simulink model "HybridControllerD2D2"  (R2017b)
settings: Solver=FixedStepDiscrete  StartTime=0.0  StopTime=inf  FixedStep=controlPeriod  RelTol=1e-3
PreLoadFcn:
  | initializeSimulation
  | initializeSCRAMNet
  | ATS_setup
values from neighbouring files (symbols this model uses):
  controlPeriod = 1/2048    (= 0.00048828125)    [initializeSCRAMNet.m]
  dofID = [1]    [initializeSimulation.m]
  lhpNode = node    [initializeSCRAMNet.m]
  MRC = [2 0.05 0.001]./10    [ATS_setup.m]
  Nl = floor(tl*sample_rate)    [ATS_setup.m]
  nTbl = 1    [initializeSCRAMNet.m]
  opfNode = node    [initializeSCRAMNet.m]
  P_range = [0.9 1.1 ... (first row only)    [ATS_setup.m]
  sample = 1/2048    (= 0.00048828125)    [ATS_setup.m]
  SN = 16    [ATS_setup.m]
  stsNode = node    [initializeSCRAMNet.m]
  Threshold = 0.01    [ATS_setup.m]
  Zden = ztag.den{1}    [ATS_setup.m]
  Znum = ztag.num{1}    [ATS_setup.m]
undefined symbols (not defined in the file or in its folder): HybridCtrlParameters, Par
libraries: simulink x14, slrtlib x13, xpcsystranlib x6
(part 2 of 2)

== system HybridControllerD2D2/xPC HC/SubSystem1/For Each Subsystem/Subsystem ==
  i : Inport
  iDelay : Inport  Port=2
  Add : Sum
  Constant1 : Constant  Value=N
  If : If  IfExpression=u1 == 0
  If Action Subsystem1 : Subsystem  TreatAsAtomicUnit=on
  If Action Subsystem2 : Subsystem  TreatAsAtomicUnit=on
  trig : Outport
  wires:
  iDelay/1 -> If/1, If Action Subsystem2/2(In2)
  If/1 -> If Action Subsystem1/Action
  If/2 -> If Action Subsystem2/Action
  If Action Subsystem1/1(Out1) -> Add/1
  If Action Subsystem2/1(Out1) -> Add/2
  Add/1 -> trig/1
  i/1 -> If Action Subsystem1/2(In2), If Action Subsystem2/1(In1)
  Constant1/1 -> If Action Subsystem1/1(In1)

== system HybridControllerD2D2/xPC HC/SubSystem1/Subsystem2/If Action Subsystem1 ==
  In1 : Inport
  In2 : Inport  Port=2
  Action Port : ActionPort  ActionType=then
  Relational Operator : RelationalOperator  Operator===  OutDataTypeStr=boolean  RndMeth=Nearest
  Out1 : Outport
  wires:
  Relational Operator/1 -> Out1/1
  In1/1 -> Relational Operator/1
  In2/1 -> Relational Operator/2

== system HybridControllerD2D2/xPC HC/SubSystem1/Subsystem2/If Action Subsystem2 ==
  In1 : Inport
  In2 : Inport  Port=2
  Action Port : ActionPort  ActionType=else
  Relational Operator : RelationalOperator  Operator===  OutDataTypeStr=boolean  RndMeth=Nearest
  Out1 : Outport
  wires:
  Relational Operator/1 -> Out1/1
  In1/1 -> Relational Operator/1
  In2/1 -> Relational Operator/2

== system HybridControllerD2D2/xPC HC/SubSystem1/For Each Subsystem/Subsystem/If Action Subsystem1 ==
  In1 : Inport
  In2 : Inport  Port=2
  Action Port : ActionPort  ActionType=then
  Relational Operator : RelationalOperator  Operator===  OutDataTypeStr=boolean  RndMeth=Nearest
  Out1 : Outport
  wires:
  Relational Operator/1 -> Out1/1
  In1/1 -> Relational Operator/1
  In2/1 -> Relational Operator/2

== system HybridControllerD2D2/xPC HC/SubSystem1/For Each Subsystem/Subsystem/If Action Subsystem2 ==
  In1 : Inport
  In2 : Inport  Port=2
  Action Port : ActionPort  ActionType=else
  Relational Operator : RelationalOperator  Operator===  OutDataTypeStr=boolean  RndMeth=Nearest
  Out1 : Outport
  wires:
  Relational Operator/1 -> Out1/1
  In1/1 -> Relational Operator/1
  In2/1 -> Relational Operator/2

== stateflow chart HybridControllerD2D2/xPC HC/Predictor-Corrector ==
  state HybridController [parallel]
    settings: executionOrder=1
    state Correct
      en: state = 0;
      en: setCurSig(comD,i/N);
      en: targLocal = targD; setNewSig(targLocal);
      en: di = min(max(diSD+1/(0.1*N)*(i-iSD),0.001),1.0);
      en: i = min(i+di,N);
      en: correctD2(comD,i/N);
      en: correctV2(comV,i/N); correctA2(comA,i/N);
      du: di = min(max(diSD+1/(0.1*N)*(i-iSD),0.001),1.0);
      du: i = min(i+di,N);
      du: correctD2(comD,i/N);
      du: correctV2(comV,i/N); correctA2(comA,i/N);
    state Predict
      en: state = 1;
      en: setCurSig(comD,1.0);
      en: i = 1; iSD = 0; diSD = 1;
      en: predictD2(comD,i/N);
      en: predictV2(comV,i/N); predictA2(comA,i/N);
      du: i++;
      du: predictD2(comD,i/N);
      du: predictV2(comV,i/N); predictA2(comA,i/N);
    state Initialize
      en: i = 0; iSD = 0; diSD = 1;
      en: initData(nDOF,dtCon,dtSim,dtInt);
      en: zeroSig(comD);
      en: zeroSig(comV);
      en: zeroSig(comA);
    state AutoSlowDown
      en: state = 2;
      en: diSD = 9-i/(0.1*N);
      en: i += diSD; iSD = i;
      en: predictD2(comD,i/N);
      en: predictV2(comV,i/N); predictA2(comA,i/N);
      du: diSD = 9-i/(0.1*N);
      du: i += diSD; iSD = i;
      du: predictD2(comD,i/N);
      du: predictV2(comV,i/N); predictA2(comA,i/N);
    Correct -> Predict [order 1] : [i>=N && flag!=1]
    (default) -> Initialize
    Initialize -> Correct : [flag==1]
    Predict -> Correct [order 2] : [flag==1]
    Predict -> AutoSlowDown [order 1] : [i>=0.8*N && flag!=1]
    AutoSlowDown -> Correct : [flag==1]
    Correct -> Correct [order 2] : [flag==1]
        | {i=0; iSD=0; diSD=1}
  data: targD input double size=nDOF+1; flag input int32; comD output double size=nDOF+1; comV output double size=nDOF+1; comA output double size=nDOF+1; state output int32; i output double; N parameter int32; nDOF parameter int32; di local double; diSD local double; iSD local double; targLocal local double size=nDOF+1; dtCon parameter double; dtSim parameter double; dtInt parameter double

== matlab function HybridControllerD2D2/ATS compensator/calculate optimal coefficients ==
  data: threshold input; par input; p_range input; MRC input; X1 input; apar output; X2 input; X3 input; Y input; dm input; prev_par input; triggeri input
function apar = fcn(threshold,par,p_range,MRC,X1,X2,X3,Y,dm,prev_par,triggeri)
%#codegen
%triggero=triggeri;
apar = [par; triggeri];

if( abs( dm ) > threshold || apar(4) )
    apar(4)=1;
    
    X = [X1 X2 X3];       
    
    temp=X\Y; 
    
    apar(1:3)=temp;
    
    if( isnan( apar(1) ) + isnan( apar(2) ) + isnan( apar(3) ) )
        apar=[par; triggeri];
    end
    
    
    % maximum change of rate
    if( abs(apar(1)-prev_par(1)) > MRC(1) )
        apar(1) = prev_par(1) + sign(apar(1)-prev_par(1))*MRC(1);
    end
    if( abs(apar(2)-prev_par(2)) > MRC(2) )
        apar(2) = prev_par(2) + sign(apar(2)-prev_par(2))*MRC(2);
    end
    if( abs(apar(3)-prev_par(3)) > MRC(3) )
        apar(3) = prev_par(3) + sign(apar(3)-prev_par(3))*MRC(3);
    end
    
    % limit of coefficients
    if( apar(1) < p_range(1,1) )
        apar(1) = p_range(1,1);
    end
    
    if( apar(1) > p_range(1,2) )
        apar(1) = p_range(1,2);
    end
    
    if( apar(2) < p_range(2,1) )
        apar(2) = p_range(2,1);
    end
    
    if( apar(2) > p_range(2,2) )
        apar(2) = p_range(2,2);
    end
    
    if( apar(3) < p_range(3,1) )
        apar(3) = p_range(3,1);
    end
    
    if( apar(3) > p_range(3,2) )
        apar(3) = p_range(3,2);
    end    
    
end

== matlab function HybridControllerD2D2/ATS compensator/compensated actuator input disp. ==
  data: apar input; x input; xd input; x2d input; ut_pred output
function ut_pred = fcn(apar,x,xd,x2d)
%#codegen

ut_pred = apar(1)*x + apar(2)*xd + apar(3)*x2d;
